simulink model "SWArchi_untitled"  (R2022b)
settings: Solver=FixedStepDiscrete  StartTime=0.0  StopTime=10.0  RelTol=1e-3
model workspace (MAT data in the model file):
  interface0 = Simulink.Bus
  interface0.Alignment = -1
  interface0.PreserveElementDimensions = 0
  interface0.Elements_internal(1) = Simulink.BusElement
  interface0.Elements_internal(1).DimensionsMode = 'Fixed'
  interface0.Elements_internal(1).SamplingMode = 'Sample based'
  interface0.Elements_internal(1).SampleTime = -1
  interface0.Elements_internal(1).Name = 'elem0'
  interface0.Elements_internal(1).DataType_internal = 'boolean'
  interface0.Elements_internal(1).Complexity = 'real'
  interface0.Elements_internal(1).Dimensions = 1
  interface0.Elements_internal(2) = Simulink.BusElement
  interface0.Elements_internal(2).DimensionsMode = 'Fixed'
  interface0.Elements_internal(2).SamplingMode = 'Sample based'
  interface0.Elements_internal(2).SampleTime = -1
  interface0.Elements_internal(2).Name = 'elem1'
  interface0.Elements_internal(2).DataType_internal = 'double'
  interface0.Elements_internal(2).Complexity = 'real'
  interface0.Elements_internal(2).Dimensions = 1
  interface0.DataScope = 'Auto'
settings Model: Creator=lcx19  LastModifiedBy=lcx19

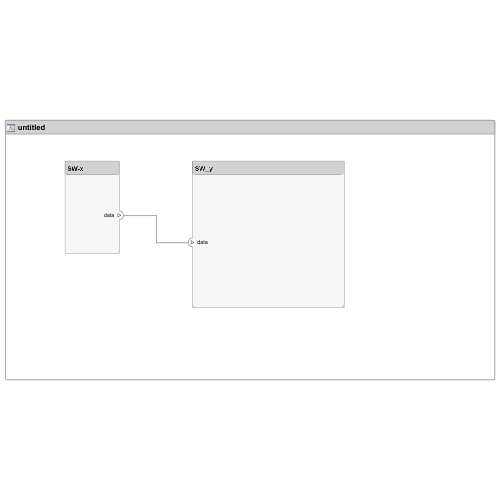
[thumbnail: Simulink's stored preview of the top-level diagram]
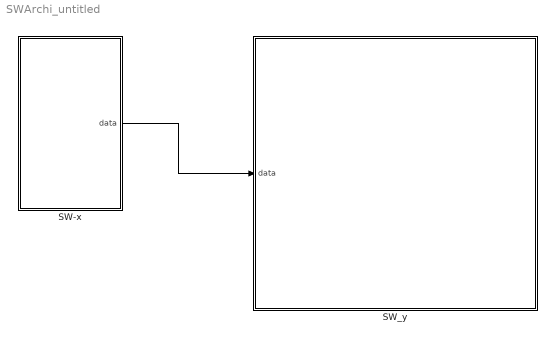
== system SWArchi_untitled ==
  SW-x : Subsystem
      settings: PortSchema="{\"entries\":[{\"content\":{\"headerSize\":26,\"margin\":15,\"minimumSpacing\":25,\"sides\":[{\"content\":{\"connectorIds\":[]},\"type\":\"ConnectorPlacement.EquallySpacedRectSide\",\"uuid\":\"db22e359-ff10-44bb-9a99-ac3b12ff4bab\"},{\"content\":{\"connectorIds\":[\"Out1\"],\"side\":\"RIGHT\"},\"type\":\"ConnectorPlacement.EquallySpacedRectSide\",\"uuid\":\"6bf61e83-7ed3-42a0-8c96-0b85b5c6bfa0\"},{\"content\":{\"connectorIds\":[],\"side\":\"TOP\"},\"type\":\"ConnectorPlacement.EquallySpacedRectSide\",\"uuid\":\"c0204a3a-7419-4482-aa3a-a0774fc2d0b0\"}]},\"type\":\"ConnectorPlacement.EquallySpacedConnector\",\"uuid\":\"d7587d40-da8e-4501-86fc-604082da4fa0\"}],\"packageUris\":[\"http://schema.mathworks.com/mf0/Connector/R2020b\"],\"version\":\"1.0\"}"
  SW_y : Subsystem
      settings: PortSchema="{\"entries\":[{\"content\":{\"headerSize\":26,\"margin\":15,\"minimumSpacing\":25,\"sides\":[{\"content\":{\"connectorIds\":[\"In1\"]},\"type\":\"ConnectorPlacement.EquallySpacedRectSide\",\"uuid\":\"db22e359-ff10-44bb-9a99-ac3b12ff4bab\"},{\"content\":{\"connectorIds\":[],\"side\":\"RIGHT\"},\"type\":\"ConnectorPlacement.EquallySpacedRectSide\",\"uuid\":\"6bf61e83-7ed3-42a0-8c96-0b85b5c6bfa0\"},{\"content\":{\"connectorIds\":[],\"side\":\"TOP\"},\"type\":\"ConnectorPlacement.EquallySpacedRectSide\",\"uuid\":\"c0204a3a-7419-4482-aa3a-a0774fc2d0b0\"}]},\"type\":\"ConnectorPlacement.EquallySpacedConnector\",\"uuid\":\"d7587d40-da8e-4501-86fc-604082da4fa0\"}],\"packageUris\":[\"http://schema.mathworks.com/mf0/Connector/R2020b\"],\"version\":\"1.0\"}"
  wires:
  SW-x/1(data) -> SW_y/1(data)

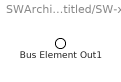
== system SWArchi_untitled/SW-x ==
  Bus Element Out1 : Outport  PortName=data

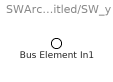
== system SWArchi_untitled/SW_y ==
  Bus Element In1 : Inport  PortName=data
